simulink model "m01_plant_model"  (R2021a)
settings: Solver=VariableStepAuto  StartTime=0.0  StopTime=10.0  RelTol=1e-3
settings Model: Creator=e102261  LastModifiedBy=s269684

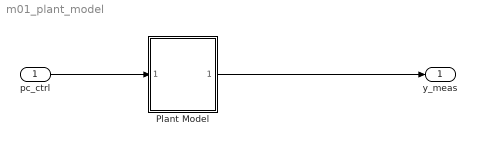
== system m01_plant_model ==
  pc_ctrl : Inport
  Plant Model : Subsystem  mask(Unreasonably Simple Plant Model){Gain_units=param.plant.Kvel, SatLimit_units=param.plant.InputSaturation, InitialPosition_deg=0}
      mask prompts: Gain_units "Gain (deg/s per input percentage unit):"; SatLimit_units "Saturation limit (input percentage units):"; InitialPosition_deg "Initial position (deg):"
      mask help: This is an unreasonably simple plant model that we came up with.
      mask Display: image('plant_image.png', 'center')
  y_meas : Outport
  wires:
  pc_ctrl/1 -> Plant Model/1(u (percent))
  Plant Model/1(y (deg)) -> y_meas/1

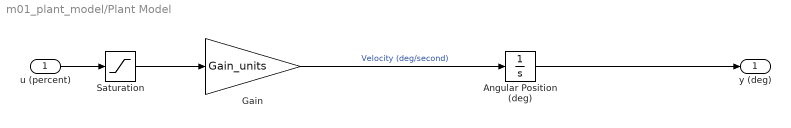
== system m01_plant_model/Plant Model ==
  u (percent) : Inport
  Angular Position (deg) : Integrator  InitialCondition=InitialPosition_deg
  Gain : Gain  Gain=Gain_units
  Saturation : Saturate  UpperLimit=SatLimit_units  LowerLimit=-SatLimit_units
      settings: AttributesFormatString=|
      | UpperLimit=%<UpperLimit>
      | LowerLimit=%<LowerLimit>
  y (deg) : Outport
  wires:
  Gain/1 -> Angular Position (deg)/1  "Velocity (deg/second)"
  Saturation/1 -> Gain/1
  Angular Position (deg)/1 -> y (deg)/1
  u (percent)/1 -> Saturation/1
